simulink model "HCW_EKF_Sim"  (R2016a)
settings: Solver=ode4  SolverMode=SingleTasking  StartTime=0  StopTime=time_end  FixedStep=time_step  MaxStep=0.1  RelTol=1e-12  AbsTol=1e-12
values from neighbouring files (symbols this model uses):
  a_chaser = 7017.9886    [FFNAV_HCW_EKF_MakeParams.m]    (also in FFNAV_HCW_PEO_Params.mat = 7500)
  a_target = 7017.9957    [FFNAV_HCW_EKF_MakeParams.m]    (also in FFNAV_HCW_PEO_Params.mat = 7500)
  AoP_chaser = AoP_target    (= -1.54915424407)    [FFNAV_HCW_EKF_MakeParams.m]    (also in FFNAV_HCW_PEO_Params.mat = 0)
  AoP_target = -88.76*pi/180    (= -1.54915424407)    [FFNAV_HCW_EKF_MakeParams.m]    (also in FFNAV_HCW_PEO_Params.mat = 0)
  e_chaser = 0.005103    [FFNAV_HCW_EKF_MakeParams.m]    (also in FFNAV_HCW_PEO_Params.mat = 0.05)
  e_target = 0.005    [FFNAV_HCW_EKF_MakeParams.m]    (also in FFNAV_HCW_PEO_Params.mat = 0)
  GPS_r_STD = (1.2*10^-3)    (= 0.0012)    [FFNAV_HCW_EKF_MakeParams.m]    (also in FFNAV_HCW_PEO_Params.mat)
  GPS_v_STD = (0.03*10^-3)    (= 3e-05)    [FFNAV_HCW_EKF_MakeParams.m]    (also in FFNAV_HCW_PEO_Params.mat)
  i_chaser = i_target    (= 0.497418836818)    [FFNAV_HCW_EKF_MakeParams.m]    (also in FFNAV_HCW_PEO_Params.mat = 0.523598775598)
  i_target = 28.5*pi/180    (= 0.497418836818)    [FFNAV_HCW_EKF_MakeParams.m]    (also in FFNAV_HCW_PEO_Params.mat = 0.523598775598)
  mu = 398600.4418    [FFNAV_HCW_EKF_MakeParams.m]    (also in FFNAV_HCW_EKFdot.m; FFNAV_HCW_PEO_Params.mat)
  n = sqrt(mu/a_target^3)    [FFNAV_HCW_EKF_MakeParams.m]    (also in FFNAV_HCW_PEO_Params.mat = 0.000972024010434)
  Q0 = [ sig2_r          0 0 0 0 0 ... (first row only)    [FFNAV_HCW_EKF_MakeParams.m]    (also in FFNAV_HCW_PEO_Params.mat = [2e-06 0 0 0 0 0 0 2e-06 0 0 0 0 ... (36 elements, 6x6)])
  R0 = [ sig2_rm                 0 0 0 0 0 ... (first row only)    [FFNAV_HCW_EKF_MakeParams.m]    (also in FFNAV_HCW_PEO_Params.mat = [0.0002 0 0 0 0 0 0 0.0002 0 0 0 0 ... (36 elements, 6x6)])
  RAAN_chaser = -1.13*pi/180    (= -0.0197222205475)    [FFNAV_HCW_EKF_MakeParams.m]    (also in FFNAV_HCW_PEO_Params.mat = 0)
  RAAN_target = 0    [FFNAV_HCW_EKF_MakeParams.m]    (also in FFNAV_HCW_PEO_Params.mat)
  theta0_chaser = 136.13*pi/180    (= 2.37591671074)    [FFNAV_HCW_EKF_MakeParams.m]    (also in FFNAV_HCW_PEO_Params.mat = 0)
  theta0_target = 135*pi/180    (= 2.35619449019)    [FFNAV_HCW_EKF_MakeParams.m]    (also in FFNAV_HCW_PEO_Params.mat = 0)
  time_step = 1    [FFNAV_HCW_EKF_RunSim.m]
undefined symbols (not defined in the file or in its folder): magnitude
settings Model: Creator=corytfraser  LastModifiedBy=Cory
settings DataIOCC: LimitDataPoints=on  SaveFormat=Array  SignalLoggingSaveFormat=ModelDataLogs
settings OptimizationCC: BlockReduction=off  BooleanDataType=off  ExpressionDepthLimit=2147483647
settings DebuggingCC: SaveWithParameterizedLinksMsg=none  UnderspecifiedInitializationDetection=Classic  MergeDetectMultiDrivingBlocksExec=none  SignalResolutionControl=TryResolveAllWithWarning  MultiTaskDSMMsg=warning  MultiTaskCondExecSysMsg=none  FcnCallInpInsideContextMsg=EnableAllAsWarning  AllowSymbolicDim=off  StateNameClashWarn=warning
settings HardwareCC: ProdBitPerPointer=32  ProdLargestAtomicFloat=None  ProdIntDivRoundTo=Undefined  ProdEndianess=Unspecified  ProdWordSize=32  ProdHWDeviceType=32-bit Generic  TargetUnknown=on
settings ModelReferenceCC: PropagateSignalLabelsOutOfModel=off
settings ConfigComp: CovModelRefEnable=Off  CovSFcnEnable=off

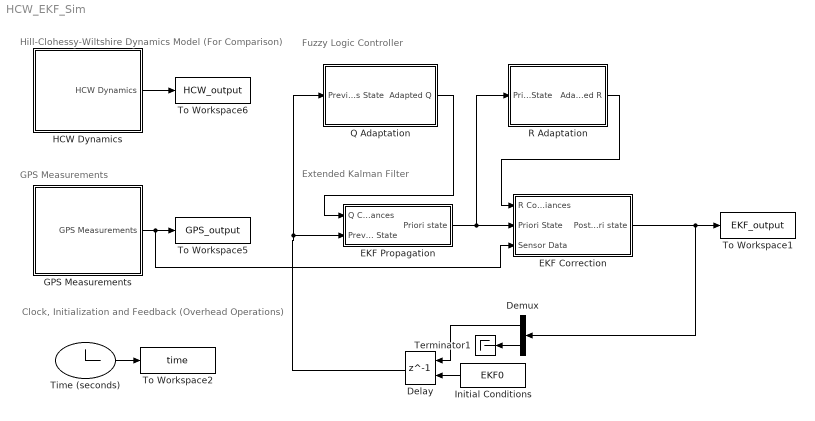
== system HCW_EKF_Sim ==
  note: Fuzzy Logic Controller
  note: Clock, Initialization and Feedback (Overhead Operations)
  note: Extended Kalman Filter
  note: GPS Measurements
  note: Hill-Clohessy-Wiltshire Dynamics Model (For Comparison)
  Delay : Delay  DelayLength=1  InitialConditionSource=Input port  InitialCondition=0  SampleTime=time_step
      settings: InputPortMap=u0,p4
  Demux : Demux  Outputs=[48 -1]
  EKF Correction : Subsystem
  EKF Propagation : Subsystem
  "GPS Measurements " : Subsystem
      mask Display: image('C:\Users\Cory\OneDrive\FFNAV Project\MATLAB Code\NERM EKF Simulation\Masks\GPS Image.jpg');
  HCW Dynamics : Subsystem
      mask Display: image('C:\Users\Cory\OneDrive\FFNAV Project\MATLAB Code\NERM EKF Simulation\Masks\Proba-3.jpg');
  Initial Conditions : FromWorkspace  VariableName=EKF0  SampleTime=time_step
  Q Adaptation : Subsystem
  "R Adaptation " : Subsystem
  Terminator1 : Terminator
  Time (seconds) : Clock
  To Workspace1 : ToWorkspace  VariableName=EKF_output  SampleTime=-1
  To Workspace2 : ToWorkspace  VariableName=time  SampleTime=-1
  To Workspace5 : ToWorkspace  VariableName=GPS_output  SampleTime=-1
  To Workspace6 : ToWorkspace  VariableName=HCW_output  SampleTime=-1
  wires:
  "GPS Measurements "/1(GPS Measurements) -> EKF Correction/3(Sensor Data), To Workspace5/1
  Time (seconds)/1 -> To Workspace2/1
  Demux/2 -> Terminator1/1
  Demux/1 -> Delay/1
  HCW Dynamics/1(HCW Dynamics) -> To Workspace6/1
  Initial Conditions/1 -> Delay/2
  EKF Propagation/1(Priori state) -> "R Adaptation "/1(Priori State), EKF Correction/2(Priori State)
  Delay/1 -> Q Adaptation/1(Previous State), EKF Propagation/2(Previous State)
  EKF Correction/1(Posteriori state) -> To Workspace1/1, Demux/1
  Q Adaptation/1(Adapted Q) -> EKF Propagation/1(Q Covariances)
  "R Adaptation "/1(Adapted R) -> EKF Correction/1(R Covariances)

== system HCW_EKF_Sim/EKF Correction ==
  R Covariances : Inport
  Priori State : Inport  Port=2
  Sensor Data : Inport  Port=3
  MATLAB Function : MATLAB Function  TreatAsAtomicUnit=on
  Posteriori state : Outport
  wires:
  MATLAB Function/1(output) -> Posteriori state/1
  Sensor Data/1 -> MATLAB Function/1(sensors)
  Priori State/1 -> MATLAB Function/2(state_pre)
  R Covariances/1 -> MATLAB Function/3(R)

== system HCW_EKF_Sim/EKF Propagation ==
  Q Covariances : Inport
  Previous State : Inport  Port=2
  Constant1 : Constant  Value=time_step
  Constant2 : Constant  Value=n
  MATLAB Function : MATLAB Function  TreatAsAtomicUnit=on
  Priori state : Outport
  wires:
  MATLAB Function/1(output) -> Priori state/1
  Previous State/1 -> MATLAB Function/3(state_pre)
  Constant1/1 -> MATLAB Function/1(time_step)
  Constant2/1 -> MATLAB Function/2(n)
  Q Covariances/1 -> MATLAB Function/4(Q)

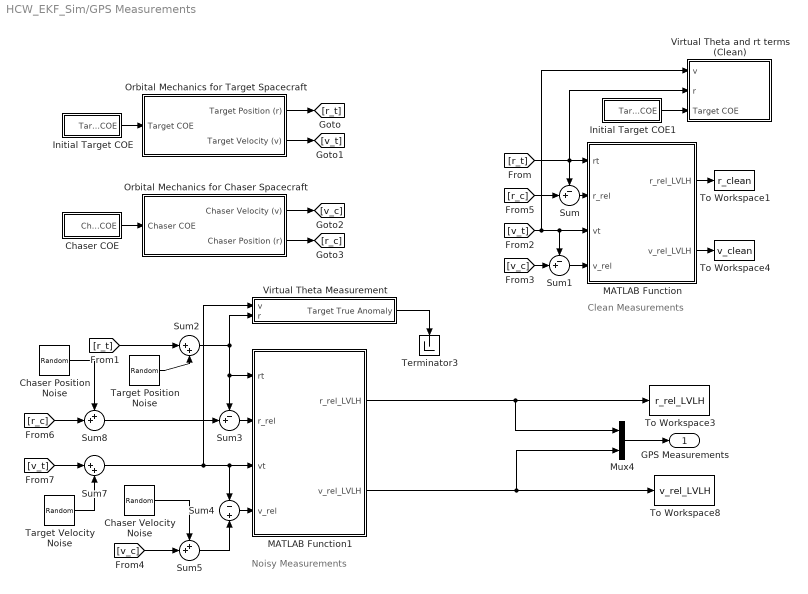
== system HCW_EKF_Sim/GPS Measurements  ==
  note: Noisy Measurements
  note: Clean Measurements
  Chaser COE : Subsystem
  Chaser Position Noise : RandomNumber  Variance=GPS_r_STD^2  Seed=1222  SampleTime=time_step
  Chaser Velocity Noise : RandomNumber  Variance=GPS_v_STD^2  Seed=99999999  SampleTime=time_step
  Initial Target COE : Subsystem
  Initial Target COE1 : Subsystem
  MATLAB Function : MATLAB Function  TreatAsAtomicUnit=on
  MATLAB Function1 : MATLAB Function  TreatAsAtomicUnit=on
  Mux4 : Mux  Inputs=2
  Orbital Mechanics for Target Spacecraft : Subsystem
  Orbital Mechanics for Chaser Spacecraft : Subsystem
  Sum : Sum  Inputs=-+|
  Sum1 : Sum  Inputs=-+|
  Sum2 : Sum  Inputs=|++
  Sum3 : Sum  Inputs=-+|
  Sum4 : Sum  Inputs=-|+
  Sum5 : Sum  Inputs=++|
  Sum7 : Sum  Inputs=|++
  Sum8 : Sum  Inputs=++|
  Target Position Noise : RandomNumber  Variance=GPS_r_STD^2  Seed=999  SampleTime=time_step
  Target Velocity Noise : RandomNumber  Variance=GPS_v_STD^2  Seed=2000  SampleTime=time_step
  Terminator3 : Terminator
  To Workspace1 : ToWorkspace  VariableName=r_clean  SampleTime=-1
  To Workspace3 : ToWorkspace  VariableName=r_rel_LVLH  SampleTime=-1
  To Workspace4 : ToWorkspace  VariableName=v_clean  SampleTime=-1
  To Workspace8 : ToWorkspace  VariableName=v_rel_LVLH  SampleTime=-1
  Virtual Theta Measurement : Subsystem
  Virtual Theta and rt terms (Clean) : Subsystem
  GPS Measurements : Outport
  wires:
  Orbital Mechanics for Target Spacecraft/1(Target Position (r)) -> [r_t]
  Sum/1 -> MATLAB Function/2(r_rel)
  Sum1/1 -> MATLAB Function/4(v_rel)
  MATLAB Function/2(v_rel_LVLH) -> To Workspace4/1
  MATLAB Function/1(r_rel_LVLH) -> To Workspace1/1
  Mux4/1 -> GPS Measurements/1
  Initial Target COE/1(Target COE) -> Orbital Mechanics for Target Spacecraft/1(Target COE)
  Chaser COE/1(Chaser COE) -> Orbital Mechanics for Chaser Spacecraft/1(Chaser COE)
  MATLAB Function1/2(v_rel_LVLH) -> To Workspace8/1, Mux4/2
  MATLAB Function1/1(r_rel_LVLH) -> Mux4/1, To Workspace3/1
  Sum7/1 -> Virtual Theta Measurement/1(v), MATLAB Function1/3(vt), Sum4/1
  Sum3/1 -> MATLAB Function1/2(r_rel)
  Sum4/1 -> MATLAB Function1/4(v_rel)
  Sum5/1 -> Sum4/2
  Sum8/1 -> Sum3/2
  [r_t] -> Virtual Theta and rt terms (Clean)/2(r), MATLAB Function/1(rt), Sum/1
  [v_t] -> Virtual Theta and rt terms (Clean)/1(v), Sum1/1, MATLAB Function/3(vt)
  [v_c] -> Sum1/2
  Orbital Mechanics for Chaser Spacecraft/1(Chaser Velocity (v)) -> [v_c]
  [r_c] -> Sum/2
  Orbital Mechanics for Chaser Spacecraft/2(Chaser Position (r)) -> [r_c]
  Orbital Mechanics for Target Spacecraft/2(Target Velocity (v)) -> [v_t]
  [r_t] -> Sum2/1
  [r_c] -> Sum8/2
  [v_t] -> Sum7/1
  [v_c] -> Sum5/2
  Sum2/1 -> MATLAB Function1/1(rt), Sum3/1, Virtual Theta Measurement/2(r)
  Chaser Position Noise/1 -> Sum8/1
  Target Position Noise/1 -> Sum2/2
  Target Velocity Noise/1 -> Sum7/2
  Chaser Velocity Noise/1 -> Sum5/1
  Initial Target COE1/1(Target COE) -> Virtual Theta and rt terms (Clean)/3(Target COE)
  Virtual Theta Measurement/1(Target True Anomaly) -> Terminator3/1

== system HCW_EKF_Sim/HCW Dynamics ==
  Demux2 : Demux  Outputs=[6 -1]
  Demux3 : Demux  Outputs=6
  HCW Equation Propagation : Subsystem
  Initial Conditions : FromWorkspace  VariableName=EKF0  SampleTime=time_step
  Mux1 : Mux  Inputs=6
  Terminator2 : Terminator
  HCW Dynamics : Outport
  wires:
  Initial Conditions/1 -> Demux2/1
  Mux1/1 -> HCW Dynamics/1
  Demux3/2 -> HCW Equation Propagation/2(y0_chaser)
  Demux3/1 -> HCW Equation Propagation/1(x0_chaser)
  HCW Equation Propagation/1(x) -> Mux1/1
  HCW Equation Propagation/2(y) -> Mux1/2
  HCW Equation Propagation/3(z) -> Mux1/3
  Demux2/1 -> Demux3/1  "Initial State Vector"
  Demux3/3 -> HCW Equation Propagation/3(z0_chaser)
  Demux3/4 -> HCW Equation Propagation/4(x_dot0_chaser)
  Demux3/5 -> HCW Equation Propagation/5(y_dot0_chaser)
  Demux3/6 -> HCW Equation Propagation/6(z_dot0_chaser)
  HCW Equation Propagation/4(x_dot) -> Mux1/4
  HCW Equation Propagation/5(y_dot) -> Mux1/5
  HCW Equation Propagation/6(z_dot) -> Mux1/6
  Demux2/2 -> Terminator2/1

== system HCW_EKF_Sim/Q Adaptation ==
  Previous State : Inport
  Constant : Constant  Value=Q0
  Constant1 : Constant  Value=Q0
  Switch: Q Adaptation On/Off : ManualSwitch  CurrentSetting=0
  Terminator : Terminator
  Adapted Q : Outport
  wires:
  Constant/1 -> Switch: Q Adaptation On/Off/2
  Switch: Q Adaptation On/Off/1 -> Adapted Q/1
  Constant1/1 -> Switch: Q Adaptation On/Off/1
  Previous State/1 -> Terminator/1

== system HCW_EKF_Sim/R Adaptation  ==
  Priori State : Inport
  Constant : Constant  Value=R0
  Constant1 : Constant  Value=R0
  Switch: R Adaptation On/Off : ManualSwitch  CurrentSetting=0
  Terminator : Terminator
  Adapted R : Outport
  wires:
  Constant/1 -> Switch: R Adaptation On/Off/2
  Switch: R Adaptation On/Off/1 -> Adapted R/1
  Priori State/1 -> Terminator/1
  Constant1/1 -> Switch: R Adaptation On/Off/1

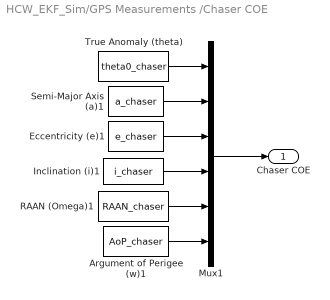
== system HCW_EKF_Sim/GPS Measurements /Chaser COE ==
  Argument of Perigee (w)1 : Constant  Value=AoP_chaser
  Eccentricity (e)1 : Constant  Value=e_chaser
  Inclination (i)1 : Constant  Value=i_chaser
  Mux1 : Mux  Inputs=6
  RAAN (Omega)1 : Constant  Value=RAAN_chaser
  Semi-Major Axis (a)1 : Constant  Value=a_chaser
  True Anomaly (theta) : Constant  Value=theta0_chaser
  Chaser COE : Outport
  wires:
  Mux1/1 -> Chaser COE/1
  Argument of Perigee (w)1/1 -> Mux1/6
  True Anomaly (theta)/1 -> Mux1/1
  Semi-Major Axis (a)1/1 -> Mux1/2
  Inclination (i)1/1 -> Mux1/4
  RAAN (Omega)1/1 -> Mux1/5
  Eccentricity (e)1/1 -> Mux1/3

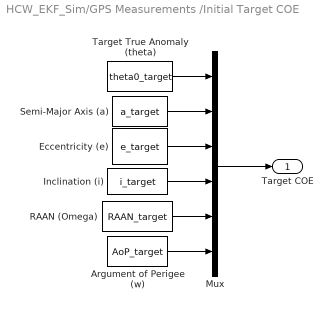
== system HCW_EKF_Sim/GPS Measurements /Initial Target COE ==
  Argument of Perigee (w) : Constant  Value=AoP_target
  Eccentricity (e) : Constant  Value=e_target
  Inclination (i) : Constant  Value=i_target
  Mux : Mux  Inputs=6
  RAAN (Omega) : Constant  Value=RAAN_target
  Semi-Major Axis (a) : Constant  Value=a_target
  Target True Anomaly (theta) : Constant  Value=theta0_target
  Target COE : Outport
  wires:
  Argument of Perigee (w)/1 -> Mux/6
  RAAN (Omega)/1 -> Mux/5
  Eccentricity (e)/1 -> Mux/3
  Semi-Major Axis (a)/1 -> Mux/2
  Target True Anomaly (theta)/1 -> Mux/1
  Inclination (i)/1 -> Mux/4
  Mux/1 -> Target COE/1

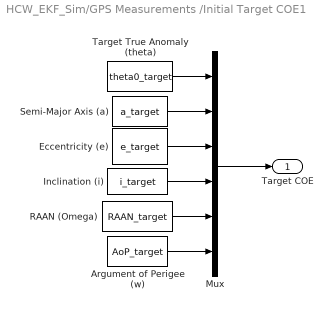
== system HCW_EKF_Sim/GPS Measurements /Initial Target COE1 ==
  Argument of Perigee (w) : Constant  Value=AoP_target
  Eccentricity (e) : Constant  Value=e_target
  Inclination (i) : Constant  Value=i_target
  Mux : Mux  Inputs=6
  RAAN (Omega) : Constant  Value=RAAN_target
  Semi-Major Axis (a) : Constant  Value=a_target
  Target True Anomaly (theta) : Constant  Value=theta0_target
  Target COE : Outport
  wires:
  Argument of Perigee (w)/1 -> Mux/6
  RAAN (Omega)/1 -> Mux/5
  Eccentricity (e)/1 -> Mux/3
  Semi-Major Axis (a)/1 -> Mux/2
  Target True Anomaly (theta)/1 -> Mux/1
  Inclination (i)/1 -> Mux/4
  Mux/1 -> Target COE/1

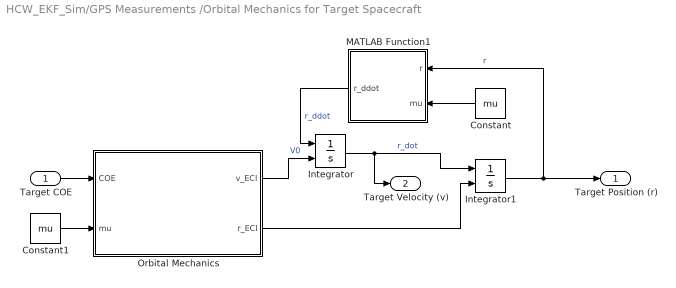
== system HCW_EKF_Sim/GPS Measurements /Orbital Mechanics for Target Spacecraft ==
  Target COE : Inport
  Constant : Constant  Value=mu
  Constant1 : Constant  Value=mu
  Integrator : Integrator  InitialConditionSource=external
  Integrator1 : Integrator  InitialConditionSource=external
  MATLAB Function1 : MATLAB Function  TreatAsAtomicUnit=on
  Orbital Mechanics : MATLAB Function  TreatAsAtomicUnit=on
  Target Position (r) : Outport
  Target Velocity (v) : Outport  Port=2
  wires:
  Integrator/1 -> Target Velocity (v)/1, Integrator1/1  "r_dot"
  MATLAB Function1/1(r_ddot) -> Integrator/1  "r_ddot"
  Integrator1/1 -> Target Position (r)/1, MATLAB Function1/1(r)  "r"
  Orbital Mechanics/2(r_ECI) -> Integrator1/2
  Orbital Mechanics/1(v_ECI) -> Integrator/2  "V0"
  Target COE/1 -> Orbital Mechanics/1(COE)
  Constant/1 -> MATLAB Function1/2(mu)
  Constant1/1 -> Orbital Mechanics/2(mu)

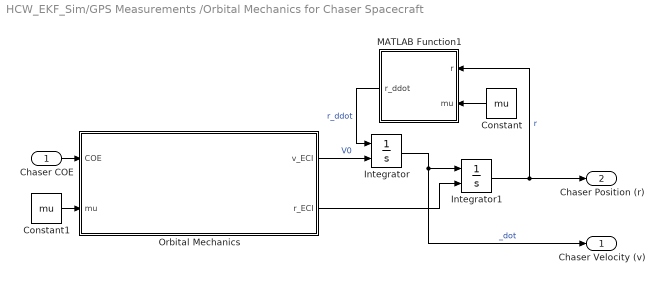
== system HCW_EKF_Sim/GPS Measurements /Orbital Mechanics for Chaser Spacecraft ==
  Chaser COE : Inport
  Constant : Constant  Value=mu
  Constant1 : Constant  Value=mu
  Integrator : Integrator  InitialConditionSource=external
  Integrator1 : Integrator  InitialConditionSource=external
  MATLAB Function1 : MATLAB Function  TreatAsAtomicUnit=on
  Orbital Mechanics : MATLAB Function  TreatAsAtomicUnit=on
  Chaser Velocity (v) : Outport
  Chaser Position (r) : Outport  Port=2
  wires:
  Integrator/1 -> Chaser Velocity (v)/1, Integrator1/1  "_dot"
  MATLAB Function1/1(r_ddot) -> Integrator/1  "r_ddot"
  Integrator1/1 -> MATLAB Function1/1(r), Chaser Position (r)/1  "r"
  Orbital Mechanics/2(r_ECI) -> Integrator1/2
  Orbital Mechanics/1(v_ECI) -> Integrator/2  "V0"
  Chaser COE/1 -> Orbital Mechanics/1(COE)
  Constant/1 -> MATLAB Function1/2(mu)
  Constant1/1 -> Orbital Mechanics/2(mu)

== system HCW_EKF_Sim/GPS Measurements /Virtual Theta Measurement ==
  v : Inport
  r : Inport  Port=2
  Constant3 : Constant  Value=theta0_target
  Integrator2 : Integrator  InitialConditionSource=external
  MATLAB Function2 : MATLAB Function  TreatAsAtomicUnit=on
  To Workspace5 : ToWorkspace  VariableName=theta_target  SampleTime=-1
  Target True Anomaly : Outport
  wires:
  r/1 -> MATLAB Function2/1(r)
  Integrator2/1 -> Target True Anomaly/1, To Workspace5/1
  MATLAB Function2/1(theta_dot) -> Integrator2/1
  Constant3/1 -> Integrator2/2
  v/1 -> MATLAB Function2/2(v)

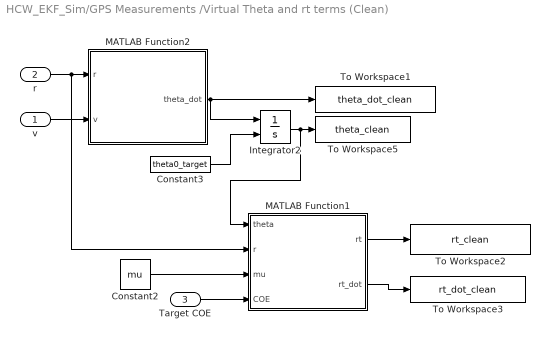
== system HCW_EKF_Sim/GPS Measurements /Virtual Theta and rt terms (Clean) ==
  v : Inport
  r : Inport  Port=2
  Target COE : Inport  Port=3
  Constant2 : Constant  Value=mu
  Constant3 : Constant  Value=theta0_target
  Integrator2 : Integrator  InitialConditionSource=external
  MATLAB Function1 : MATLAB Function  TreatAsAtomicUnit=on
  MATLAB Function2 : MATLAB Function  TreatAsAtomicUnit=on
  To Workspace1 : ToWorkspace  VariableName=theta_dot_clean  SampleTime=-1
  To Workspace2 : ToWorkspace  VariableName=rt_clean  SampleTime=-1
  To Workspace3 : ToWorkspace  VariableName=rt_dot_clean  SampleTime=-1
  To Workspace5 : ToWorkspace  VariableName=theta_clean  SampleTime=-1
  wires:
  r/1 -> MATLAB Function1/2(r), MATLAB Function2/1(r)
  Integrator2/1 -> MATLAB Function1/1(theta), To Workspace5/1
  MATLAB Function2/1(theta_dot) -> Integrator2/1, To Workspace1/1
  Constant3/1 -> Integrator2/2
  v/1 -> MATLAB Function2/2(v)
  MATLAB Function1/1(rt) -> To Workspace2/1
  MATLAB Function1/2(rt_dot) -> To Workspace3/1
  Target COE/1 -> MATLAB Function1/4(COE)
  Constant2/1 -> MATLAB Function1/3(mu)

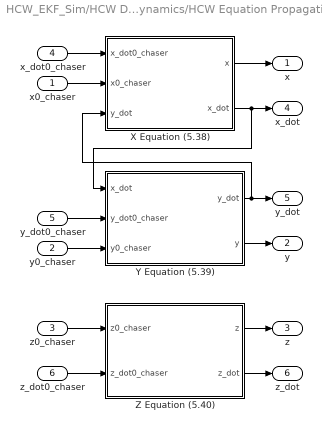
== system HCW_EKF_Sim/HCW Dynamics/HCW Equation Propagation ==
  x0_chaser : Inport
  y0_chaser : Inport  Port=2
  z0_chaser : Inport  Port=3
  x_dot0_chaser : Inport  Port=4
  y_dot0_chaser : Inport  Port=5
  z_dot0_chaser : Inport  Port=6
  X Equation (5.38) : Subsystem
  Y Equation (5.39) : Subsystem
  Z Equation (5.40) : Subsystem
  x : Outport
  y : Outport  Port=2
  z : Outport  Port=3
  x_dot : Outport  Port=4
  y_dot : Outport  Port=5
  z_dot : Outport  Port=6
  wires:
  Y Equation (5.39)/1(y_dot) -> X Equation (5.38)/3(y_dot), y_dot/1
  X Equation (5.38)/2(x_dot) -> Y Equation (5.39)/1(x_dot), x_dot/1
  X Equation (5.38)/1(x) -> x/1
  Y Equation (5.39)/2(y) -> y/1
  Z Equation (5.40)/1(z) -> z/1
  y_dot0_chaser/1 -> Y Equation (5.39)/2(y_dot0_chaser)
  y0_chaser/1 -> Y Equation (5.39)/3(y0_chaser)
  x0_chaser/1 -> X Equation (5.38)/2(x0_chaser)
  x_dot0_chaser/1 -> X Equation (5.38)/1(x_dot0_chaser)
  z0_chaser/1 -> Z Equation (5.40)/1(z0_chaser)
  z_dot0_chaser/1 -> Z Equation (5.40)/2(z_dot0_chaser)
  Z Equation (5.40)/2(z_dot) -> z_dot/1

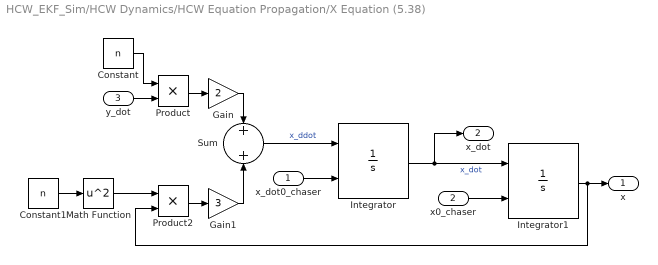
== system HCW_EKF_Sim/HCW Dynamics/HCW Equation Propagation/X Equation (5.38) ==
  x_dot0_chaser : Inport
  x0_chaser : Inport  Port=2
  y_dot : Inport  Port=3
  Constant : Constant  Value=n
  Constant1 : Constant  Value=n
  Gain : Gain  Gain=2
  Gain1 : Gain  Gain=3
  Integrator : Integrator  InitialConditionSource=external
  Integrator1 : Integrator  InitialConditionSource=external
  Math Function : Math  Operator=square  SaturateOnIntegerOverflow=on
  Product : Product
  Product2 : Product
  Sum : Sum
  x : Outport
  x_dot : Outport  Port=2
  wires:
  Sum/1 -> Integrator/1  "x_ddot"
  Integrator/1 -> Integrator1/1, x_dot/1  "x_dot"
  x_dot0_chaser/1 -> Integrator/2
  x0_chaser/1 -> Integrator1/2
  Integrator1/1 -> Product2/2, x/1
  Product/1 -> Gain/1
  y_dot/1 -> Product/2
  Math Function/1 -> Product2/1
  Constant/1 -> Product/1
  Constant1/1 -> Math Function/1
  Product2/1 -> Gain1/1
  Gain/1 -> Sum/1
  Gain1/1 -> Sum/2

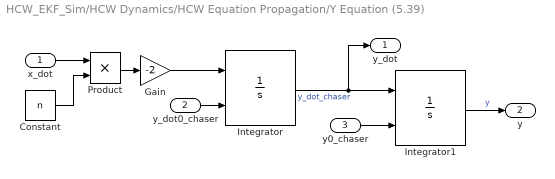
== system HCW_EKF_Sim/HCW Dynamics/HCW Equation Propagation/Y Equation (5.39) ==
  x_dot : Inport
  y_dot0_chaser : Inport  Port=2
  y0_chaser : Inport  Port=3
  Constant : Constant  Value=n
  Gain : Gain  Gain=-2
  Integrator : Integrator  InitialConditionSource=external
  Integrator1 : Integrator  InitialConditionSource=external
  Product : Product
  y_dot : Outport
  y : Outport  Port=2
  wires:
  y_dot0_chaser/1 -> Integrator/2
  y0_chaser/1 -> Integrator1/2
  Integrator/1 -> y_dot/1, Integrator1/1  "y_dot_chaser"
  Integrator1/1 -> y/1  "y"
  Product/1 -> Gain/1
  x_dot/1 -> Product/1
  Constant/1 -> Product/2
  Gain/1 -> Integrator/1

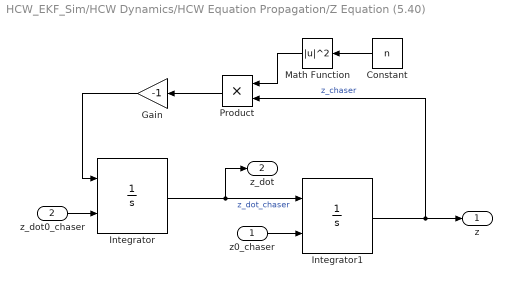
== system HCW_EKF_Sim/HCW Dynamics/HCW Equation Propagation/Z Equation (5.40) ==
  z0_chaser : Inport
  z_dot0_chaser : Inport  Port=2
  Constant : Constant  Value=n
  Gain : Gain  Gain=-1
  Integrator : Integrator  InitialConditionSource=external
  Integrator1 : Integrator  InitialConditionSource=external
  Math Function : Math  Operator=magnitude^2  SaturateOnIntegerOverflow=on
  Product : Product
  z : Outport
  z_dot : Outport  Port=2
  wires:
  Integrator/1 -> z_dot/1, Integrator1/1  "z_dot_chaser"
  Integrator1/1 -> Product/2, z/1  "z_chaser"
  Gain/1 -> Integrator/1
  z_dot0_chaser/1 -> Integrator/2
  z0_chaser/1 -> Integrator1/2
  Product/1 -> Gain/1
  Math Function/1 -> Product/1
  Constant/1 -> Math Function/1

== matlab function HCW_EKF_Sim/GPS Measurements /Orbital Mechanics for Target Spacecraft/MATLAB Function1 ==
  data: r input; r_ddot output; mu input
function r_ddot = r_ddot(r, mu)
% ========================================================================
% Description: This function calculates -mu/r^3 *r to propagate the radius
% vector of the orbital motion

r_ddot = -(mu/(norm(r))^3)*r;

end
% ========================================================================

== matlab function HCW_EKF_Sim/GPS Measurements /Orbital Mechanics for Target Spacecraft/Orbital Mechanics ==
  data: v_ECI output; COE input; r_ECI output; mu input
 function [v_ECI,r_ECI] = Orb_Mech(COE, mu)
% ========================================================================
% Description: This funciton calculates the initial r and v vectors, 
% given the provided classiclal orbital elements defined in the
% initialization of the simulation.

%%========================================================================
%Extract COE values
theta       = COE(1);
a           = COE(2);
e           = COE(3);
i           = COE(4);
RAAN        = COE(5);
w           = COE(6);

%%========================================================================
r   = a*(1-e^2)/(1+e*cos(theta));                               %Defining the radius (Eq. 2.32)
p   = a*(1-e^2);                                                %Defining the semilatus rectum (Eq. 2.31)
r_P = [r*cos(theta) r*sin(theta) 0]';                           %(r in perifocal frame - Eq. 2.86) 
v_P = [-sqrt(mu/p)*sin(theta) sqrt(mu/p)*(e+cos(theta)) 0]';    %(v in perifocal frame - Eq. 2.87)

%Rotation Matrix from P to ECI Frame
C_IP = [    cos(RAAN)*cos(w)-sin(RAAN)*cos(i)*sin(w) -cos(RAAN)*sin(w)-sin(RAAN)*cos(i)*cos(w) sin(RAAN)*sin(i);
            sin(RAAN)*cos(w)+cos(RAAN)*cos(i)*sin(w) -sin(RAAN)*sin(w)+cos(RAAN)*cos(i)*cos(w) -cos(RAAN)*sin(i);
                        sin(i)*sin(w)                            sin(i)*cos(w)                       cos(i)  ];

%Definition of ECI Frame
x_ECI   = [1 0 0];
y_ECI   = [0 1 0];
z_ECI   = [0 0 1];
F_ECI   = [x_ECI; y_ECI; z_ECI]; %Reference Frame ECI

%r and v vectors in ECI Frame
r_ECI   = F_ECI*C_IP*r_P;
v_ECI   = F_ECI*C_IP*v_P;

%z_vec_ECI  = cross(r_ECI, v_ECI)/norm(cross(r_ECI, v_ECI));    %Check orientation of z vector
%X_ECI      = [r_ECI v_ECI]';                                   %State Vector in ECI components (Eq. 2.82)

r_mag = norm(r_ECI);
r_hat = r_ECI/r_mag;

end
% ========================================================================

== matlab function HCW_EKF_Sim/GPS Measurements /Orbital Mechanics for Chaser Spacecraft/MATLAB Function1 ==
  data: r input; r_ddot output; mu input
function r_ddot = r_ddot(r, mu)
% ========================================================================
% Description: This function calculates -mu/r^3 *r to propagate the radius
% vector of the orbital motion

r_ddot = -(mu/(norm(r))^3)*r;

end
% ========================================================================

== matlab function HCW_EKF_Sim/GPS Measurements /Orbital Mechanics for Chaser Spacecraft/Orbital Mechanics ==
  data: v_ECI output; COE input; r_ECI output; mu input
function [v_ECI,r_ECI] = Orb_Mech(COE, mu)
% ========================================================================
% Description: This funciton calculates the initial r and v vectors, 
% given the provided classiclal orbital elements defined in the
% initialization of the simulation.

%%========================================================================
%Extract COE values
theta       = COE(1);
a           = COE(2);
e           = COE(3);
i           = COE(4);
RAAN        = COE(5);
w           = COE(6);

%%========================================================================
r   = a*(1-e^2)/(1+e*cos(theta));                               %Defining the radius (Eq. 2.32)
p   = a*(1-e^2);                                                %Defining the semilatus rectum (Eq. 31)
r_P = [r*cos(theta) r*sin(theta) 0]';                           %(r in perifocal frame - Eq. 2.86) 
v_P = [-sqrt(mu/p)*sin(theta) sqrt(mu/p)*(e+cos(theta)) 0]';    %(v in perifocal frame - Eq. 2.87)

%Rotation Matrix from P to ECI Frame
C_IP = [    cos(RAAN)*cos(w)-sin(RAAN)*cos(i)*sin(w) -cos(RAAN)*sin(w)-sin(RAAN)*cos(i)*cos(w) sin(RAAN)*sin(i);
            sin(RAAN)*cos(w)+cos(RAAN)*cos(i)*sin(w) -sin(RAAN)*sin(w)+cos(RAAN)*cos(i)*cos(w) -cos(RAAN)*sin(i);
                        sin(i)*sin(w)                            sin(i)*cos(w)                       cos(i)  ];

%Definition of ECI Frame
x_ECI   = [1 0 0];
y_ECI   = [0 1 0];
z_ECI   = [0 0 1];
F_ECI   = [x_ECI; y_ECI; z_ECI]; %Reference Frame ECI

%r and v vectors in ECI Frame
r_ECI   = F_ECI*C_IP*r_P;
v_ECI   = F_ECI*C_IP*v_P;

%z_vec_ECI  = cross(r_ECI, v_ECI)/norm(cross(r_ECI, v_ECI));    %Check orientation of z vector
%X_ECI      = [r_ECI v_ECI]';                                   %State Vector in ECI components (Eq. 2.82)

r_mag = norm(r_ECI);
r_hat = r_ECI/r_mag;

end
% ========================================================================

== matlab function HCW_EKF_Sim/GPS Measurements /MATLAB Function ==
  data: rt input; r_rel input; vt input; r_rel_LVLH output; v_rel input; v_rel_LVLH output
 function [r_rel_LVLH, v_rel_LVLH] = To_LVLH(rt, r_rel, vt, v_rel)
% =========================================================================
% Description: This function converts the relative r and v from ECI Frame
% to LVLH Frame by applying the appropriate rotation matrices.
% =========================================================================
%Determine unit vectors for LVLH Frame
Lx      = rt/norm(rt);
Lz      = cross(rt, vt)/norm(cross(rt, vt));
Ly      = cross(Lz, Lx);

%Align unit vectors into rows
Lx      = Lx';
Ly      = Ly';
Lz      = Lz';

%Arranging vectrix for LVLH Frame
F_LVLH  = [ Lx      
            Ly
            Lz ];

%ECI Frame is defined as such
F_ECI   = [ 1 0 0 
            0 1 0
            0 0 1 ];
     
%Compute roration matrix - ECI to LVLH
C_LI    = F_LVLH*F_ECI';

%Computing relative velocity in LVLH frame, accounting for rotation 
omega =  cross(rt,vt)/norm(rt)^2;
v_rel = v_rel - cross(omega,r_rel);

%Apply rotation to obtain relative LVLH parameters
r_rel_LVLH = C_LI*r_rel; 
v_rel_LVLH = C_LI*v_rel;

end
% =========================================================================

== matlab function HCW_EKF_Sim/GPS Measurements /Virtual Theta Measurement/MATLAB Function2 ==
  data: r input; v input; theta_dot output
function theta_dot  = theta_dot(r, v)
% ========================================================================
% Description: This function calculates h/r^2 to propagate the true 
% anomaly of the target spacecraft
rt = norm(r);
h = norm(cross(r,v));
theta_dot = h/rt^2;

end
% ========================================================================

== matlab function HCW_EKF_Sim/GPS Measurements /MATLAB Function1 ==
  data: rt input; r_rel input; vt input; r_rel_LVLH output; v_rel input; v_rel_LVLH output
 function [r_rel_LVLH, v_rel_LVLH] = To_LVLH(rt, r_rel, vt, v_rel)
% =========================================================================
% Description: This function converts the relative r and v from ECI Frame
% to LVLH Frame by applying the appropriate rotation matrices.
% =========================================================================
%Determine unit vectors for LVLH Frame
Lx      = rt/norm(rt);
Lz      = cross(rt, vt)/norm(cross(rt, vt));
Ly      = cross(Lz, Lx);

%Align unit vectors into rows
Lx      = Lx';
Ly      = Ly';
Lz      = Lz';

%Arranging vectrix for LVLH Frame
F_LVLH  = [ Lx
            Ly
            Lz ];

%ECI Frame is defined as such
F_ECI   = [ 1 0 0 
            0 1 0
            0 0 1 ];
     
%Compute roration matrix - ECI to LVLH
C_LI    = F_LVLH*F_ECI';

%Computing relative velocity in LVLH frame, accounting for rotation 
omega =  cross(rt,vt)/norm(rt)^2;
v_rel = v_rel - cross(omega,r_rel);

%Apply rotation to obtain relative LVLH parameters
r_rel_LVLH = C_LI*r_rel; 
v_rel_LVLH = C_LI*v_rel;

end
% =========================================================================

== matlab function HCW_EKF_Sim/GPS Measurements /Virtual Theta and rt terms (Clean)/MATLAB Function2 ==
  data: r input; v input; theta_dot output
function theta_dot  = theta_dot(r, v)
% ========================================================================
% Description: This function calculates h/r^2 to propagate the true 
% anomaly of the target spacecraft
rt = norm(r);
h = norm(cross(r,v));
theta_dot = h/rt^2;

end
% ========================================================================

== matlab function HCW_EKF_Sim/EKF Correction/MATLAB Function ==
  data: sensors input; state_pre input; output output; R input
 function output = USE_EKF_Correction(sensors, state_pre, R)
%% USE_EKF ===============================================================
% ========================================================================
% Description: This function calls the FFNAV_EKF Function, which completes 
% the covariance propagation and correction phases of the EKF algorithm. 
% The output is then passed back to the simulink model.

output = zeros(90,1);
output = FFNAV_HCW_EKF_Correction(sensors, state_pre, R);
end
% ========================================================================

== matlab function HCW_EKF_Sim/EKF Propagation/MATLAB Function ==
  data: time_step input; n input; state_pre input; output output; Q input
 function output = USE_EKF_Propagation(time_step, n, state_pre, Q)
%% USE_EKF ===============================================================
% ========================================================================
% Description: This function calls the FFNAV_EKF Function, which completes 
% the covariance propagation and correction phases of the EKF algorithm. 
% The output is then passed back to the simulink model.

output = zeros(42,1);
output = FFNAV_HCW_EKF_Propagation(time_step, state_pre, n, Q);
end
% ========================================================================

== matlab function HCW_EKF_Sim/GPS Measurements /Virtual Theta and rt terms (Clean)/MATLAB Function1 ==
  data: theta input; r input; rt output; rt_dot output; mu input; COE input
function [rt, rt_dot]  = rt_rtdot(theta, r, mu, COE)
% ========================================================================
% Description: This function calculates h/r^2 to propagate the true 
% anomaly of the target spacecraft

theta0       = COE(1);
a           = COE(2);
e           = COE(3);
i           = COE(4);
RAAN        = COE(5);
w           = COE(6);

rt      = norm(r);
p       = a*(1-e^2);
rt_dot  = sqrt(mu/p)*e*sin(theta);

end
% ========================================================================
